simulink model "estimation"  (R2014a)
settings: Solver=ode1  StartTime=0.0  StopTime=20  FixedStep=Ts  RelTol=1e-3
InitFcn:
  | estimation_initfcn
values from neighbouring files (symbols this model uses):
  c = [x y z]'    [estimation_initfcn.m]
  I_p = (I_q+m*(c'*c*eye(3)-c*c'))'    [estimation_initfcn.m]
  m = 2    [estimation_initfcn.m]
settings Model: Creator=wirnshofer  LastModifiedBy=bschmidt
settings DebuggingCC: MergeDetectMultiDrivingBlocksExec=error

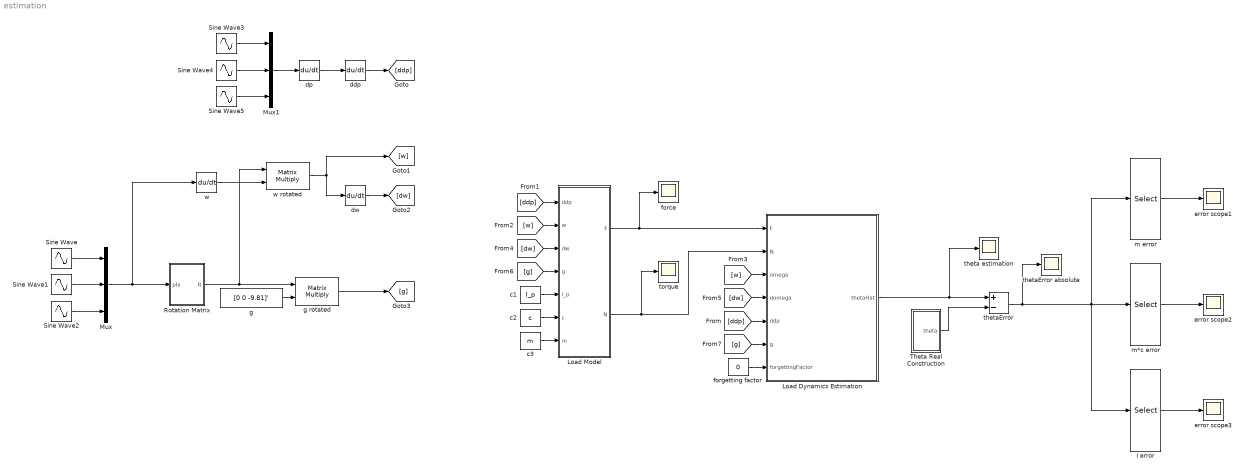
== system estimation ==
  I error : Selector  InputPortWidth=10  Indices=[5:10]
  Load Dynamics Estimation : MATLAB Function  TreatAsAtomicUnit=on
  Load Model : MATLAB Function  TreatAsAtomicUnit=on
  Mux : Mux  Inputs=3
  Mux1 : Mux  Inputs=3
  Rotation Matrix : MATLAB Function  TreatAsAtomicUnit=on
  Sine Wave : Sin  Frequency=2  SampleTime=0
  Sine Wave1 : Sin  Frequency=3  SampleTime=0
  Sine Wave2 : Sin  Frequency=4  SampleTime=0
  Sine Wave3 : Sin  Frequency=5  SampleTime=0
  Sine Wave4 : Sin  Frequency=6  SampleTime=0
  Sine Wave5 : Sin  Frequency=7  SampleTime=0
  Theta Real Construction : Subsystem
  c1 : Constant  Value=I_p
  c2 : Constant  Value=c
  c3 : Constant  Value=m
  ddp : Derivative
  dp : Derivative
  dw : Derivative
  error scope1 : Scope
      settings: ShowLegends=on  TimeRange=20  YMin=-0.0001501181625771192  YMax=9.095565469484932e-05  SaveName=thetaError
  error scope2 : Scope
      settings: ShowLegends=on  TimeRange=20  YMin=-0.0001501181625771192  YMax=9.095565469484932e-05  SaveName=thetaError5
  error scope3 : Scope
      settings: ShowLegends=on  TimeRange=20  YMin=-0.002044113384259428  YMax=0.001899055514507558  SaveName=thetaError6
  force : Scope
      settings: ShowLegends=on  YMin=-20  YMax=0  SaveName=thetaError3
  forgetting factor : Constant  Value=0
  g : Constant  Value=[0 0 -9.81]'
  g rotated : Product  Multiplication=Matrix(*)
  m error : Selector  InputPortWidth=10  Indices=[1]
  m*c error : Selector  InputPortWidth=10  Indices=[2:4]
  theta estimation : Scope
      settings: ShowLegends=on  YMin=-0.5  YMax=8.5  SaveName=thetaError2
  thetaError : Sum  Inputs=+-
  thetaError absolute : Scope
      settings: ShowLegends=on  TimeRange=20  YMin=-0.0009991012166885793  YMax=0.001009966988737202  SaveName=thetaError1
  torque : Scope
      settings: ShowLegends=on  YMin=-0.5  YMax=8.5  SaveName=thetaError4
  w : Derivative
  w rotated : Product  Multiplication=Matrix(*)
  wires:
  g/1 -> g rotated/2
  forgetting factor/1 -> Load Dynamics Estimation/7(forgettingFactor)
  Load Dynamics Estimation/1(thetaHat) -> theta estimation/1, thetaError/1
  Theta Real Construction/1(theta) -> thetaError/2
  thetaError/1 -> thetaError absolute/1, I error/1, m*c error/1, m error/1
  Load Model/1(F) -> Load Dynamics Estimation/1(F), force/1
  Mux/1 -> w/1, Rotation Matrix/1(phi)
  Rotation Matrix/1(R) -> w rotated/1, g rotated/1
  Mux1/1 -> dp/1
  w rotated/1 -> dw/1, [w]
  dw/1 -> [dw]
  Load Model/2(N) -> torque/1, Load Dynamics Estimation/2(N)
  Sine Wave/1 -> Mux/1
  Sine Wave1/1 -> Mux/2
  Sine Wave2/1 -> Mux/3
  w/1 -> w rotated/2
  Sine Wave3/1 -> Mux1/1
  Sine Wave4/1 -> Mux1/2
  Sine Wave5/1 -> Mux1/3
  dp/1 -> ddp/1
  m error/1 -> error scope1/1
  m*c error/1 -> error scope2/1
  I error/1 -> error scope3/1
  c1/1 -> Load Model/5(I_p)
  c2/1 -> Load Model/6(c)
  c3/1 -> Load Model/7(m)
  ddp/1 -> [ddp]
  [ddp] -> Load Dynamics Estimation/5(ddp)
  [ddp] -> Load Model/1(ddp)
  [w] -> Load Dynamics Estimation/3(omega)
  [dw] -> Load Model/3(dw)
  [w] -> Load Model/2(w)
  [dw] -> Load Dynamics Estimation/4(domega)
  g rotated/1 -> [g]
  [g] -> Load Model/4(g)
  [g] -> Load Dynamics Estimation/6(g)

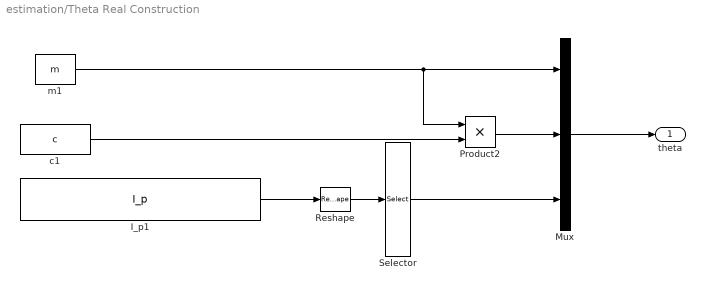
== system estimation/Theta Real Construction ==
  I_p1 : Constant  Value=I_p  VectorParams1D=off
  Mux : Mux  Inputs=3
  Product2 : Product
  Reshape : Reshape
  Selector : Selector  InputPortWidth=9  Indices=[1 2 3 5 6 9]
  c1 : Constant  Value=c
  m1 : Constant  Value=m
  theta : Outport
  wires:
  m1/1 -> Product2/1, Mux/1
  c1/1 -> Product2/2
  Product2/1 -> Mux/2
  Mux/1 -> theta/1
  I_p1/1 -> Reshape/1
  Reshape/1 -> Selector/1
  Selector/1 -> Mux/3

== matlab function estimation/Load Dynamics Estimation ==
  data: F input; thetaHat output; N input; omega input; domega input; ddp input; g input; forgettingFactor input
function thetaHat = fcn(F,N,omega,domega,ddp,g,forgettingFactor)
    thetaHat = estimationOneGraspingPoint(F,N,omega,domega,ddp,g,forgettingFactor,0);
end

== matlab function estimation/Load Model ==
  data: ddp input; F output; w input; dw input; g input; N output; I_p input; c input; m input
function [F, N] = fcn(ddp, w, dw, g, I_p, c, m)
% all variables except ddp are in the sensor frame, including g

F = m*ddp + m*g + cross(dw, m*c) + cross(w, cross(w, m*c));
N = I_p*dw + cross(w, I_p*w) + cross(m*c, ddp) + cross(m*c, g);

== matlab function estimation/Rotation Matrix ==
  data: phi input; R output
function R = fcn(phi)
    R = createRotationMatrix(phi);
end
